simulink model "sf_loop_scheduler"  (R2017b)
settings: Solver=FixedStepDiscrete  StartTime=0.0  StopTime=10  RelTol=1e-3  EnableMultiTasking=on
model workspace (MAT data in the model file):
  deltat = 0.001
settings Model: Creator=The MathWorks, Inc.  LastModifiedBy=The MathWorks, Inc.
settings SolverCC: InsertRTBMode=Auto
settings DataIOCC: LimitDataPoints=on  SaveFormat=Array
settings OptimizationCC: ExpressionDepthLimit=2147483647  InitFltsAndDblsToZero=on  LifeSpan=inf
settings DebuggingCC: SaveWithParameterizedLinksMsg=none  UnderspecifiedInitializationDetection=Classic  MergeDetectMultiDrivingBlocksExec=none  SignalResolutionControl=TryResolveAllWithWarning  InheritedTsInSrcMsg=none  MultiTaskDSMMsg=warning  MultiTaskCondExecSysMsg=none  FcnCallInpInsideContextMsg=warning  StateNameClashWarn=warning  StrictBusMsg=None  SFUnexpectedBacktrackingDiag=warning  SFNoUnconditionalDefaultTransitionDiag=warning  SFExecutionAtInitializationDiag=none
settings HardwareCC: ProdBitPerPointer=32  ProdBitPerSizeT=32  ProdBitPerPtrDiffT=32  ProdLargestAtomicFloat=None  ProdIntDivRoundTo=Undefined  ProdEndianess=Unspecified  ProdWordSize=32  ProdHWDeviceType=32-bit Generic
settings ModelReferenceCC: PropagateSignalLabelsOutOfModel=off
settings SFSimCC: SFSimEcho=off  SimParseCustomCode=off
settings CodeAppCC: StateflowObjectComments=on
settings GRTTargetCC: TargetFcnLib=ansi_tfl_tmw.mat  TargetLangStandard=C89/C90 (ANSI)  GeneratePreprocessorConditionals=Disable all  CombineOutputUpdateFcns=off  GRTInterface=on
settings ConfigComp: CovMetricSettings=dw  CovHtmlReporting=on  CovSaveCumulativeToWorkspaceVar=on  CovSaveSingleToWorkspaceVar=on  CovExternalEMLEnable=off  CovSFcnEnable=off

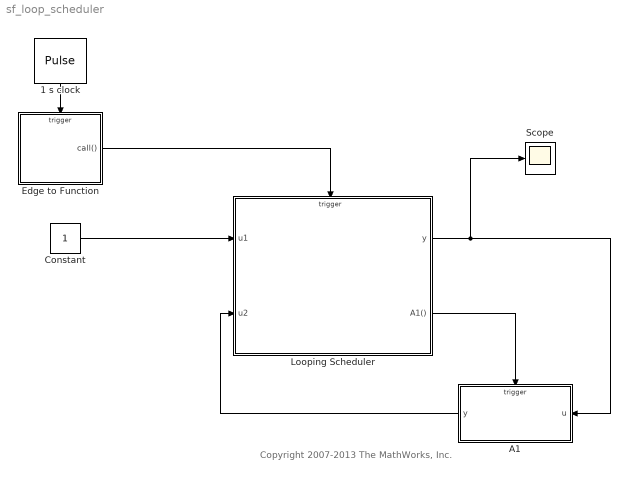
== system sf_loop_scheduler ==
  note: Copyright 2007-2013 The MathWorks, Inc.
  1 s clock : DiscretePulseGenerator  PulseType=Time based  Period=1  PulseWidth=10
  A1 : Subsystem  TreatAsAtomicUnit=on
  Constant : Constant
  "Edge to Function " : Stateflow chart  TreatAsAtomicUnit=on
  Looping Scheduler : Stateflow chart  TreatAsAtomicUnit=on
  Scope : Scope
  wires:
  Looping Scheduler/1(y) -> A1/1(u), Scope/1
  Looping Scheduler/2(A1()) -> A1/Trigger
  A1/1(y) -> Looping Scheduler/2(u2)
  Constant/1 -> Looping Scheduler/1(u1)
  1 s clock/1 -> "Edge to Function "/Trigger
  "Edge to Function "/1(call()) -> Looping Scheduler/Trigger

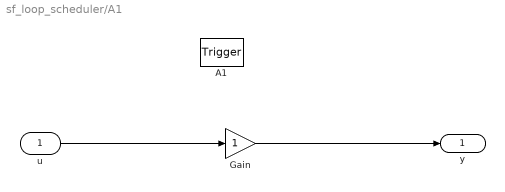
== system sf_loop_scheduler/A1 ==
  u : Inport
  A1 : TriggerPort  TriggerType=function-call  VariantControl=Variant
  Gain : Gain
  y : Outport
  wires:
  u/1 -> Gain/1
  Gain/1 -> y/1

== stateflow chart sf_loop_scheduler/Looping Scheduler ==
  (default) -> (junction 5) : {i=1;}
  (junction 6) -> (junction 5) [order 1] : [i<=10]
      | {
      |  y = u1+u2;
      | send(A1);
      | i++;
      | }
  (junction 5) -> (junction 6)
  (junction 6) -> (junction 7) [order 2] : // done
  data: y output double; u1 input; u2 input; i local uint32
  events: A1 output FUNCTION_CALL_EVENT; call input FUNCTION_CALL_EVENT

== stateflow chart sf_loop_scheduler/Edge to Function  ==
  (default) -> (junction 2) : {call;}
  events: edge input RISING_EDGE_EVENT; call output FUNCTION_CALL_EVENT
